simulink model "robot_capteur_etu"  (R2022a)
settings: Solver=VariableStepAuto  StartTime=0.0  StopTime=10.0  RelTol=1e-3
values from neighbouring files (symbols this model uses):
  K = -place(A, B, poles)    [matrices.m]    (also in sensibilite_parametre.m = [0.6700, 19.9053, 1.0747, 1.9614]; simu_robot_etu.m = [0.6700, 19.9055, 1.0747, 1.9614])
  ue = 0    [sensibilite_parametre.m]    (also in simu_robot_etu.m)
  x0 = [0 pi/10 0 0]'    [sensibilite_parametre.m]    (also in simu_robot_etu.m)
  xe = [0 0 0 0]'    [sensibilite_parametre.m]    (also in simu_robot_etu.m)
settings Model: Creator=nauchere  LastModifiedBy=nauchere

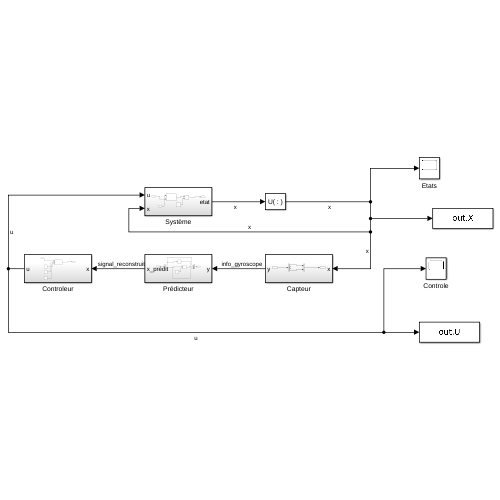
[thumbnail: Simulink's stored preview of the top-level diagram]
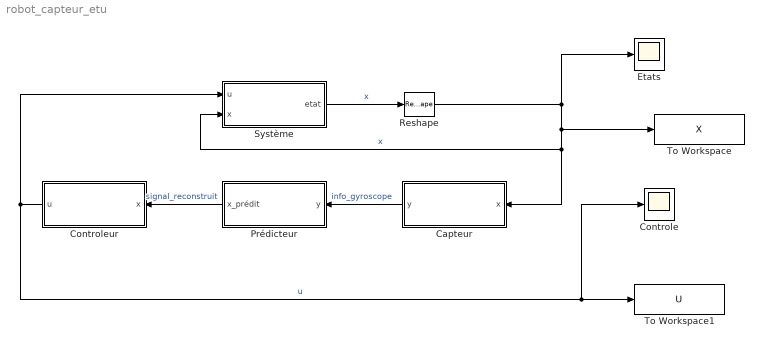
== system robot_capteur_etu ==
  Capteur : Subsystem
  Controle : Scope
  Controleur : Subsystem
  Etats : Scope
  Prédicteur : Subsystem
  Reshape : Reshape
  Système : Subsystem
  To Workspace : ToWorkspace  VariableName=X  SaveFormat=Timeseries  SampleTime=-1
  To Workspace1 : ToWorkspace  VariableName=U  SaveFormat=Timeseries  SampleTime=-1
  wires:
  Controleur/1(u) -> Système/1(u), Controle/1, To Workspace1/1  "u"
  Prédicteur/1(x_prédit) -> Controleur/1(x)  "signal_reconstruit"
  Capteur/1(y) -> Prédicteur/1(y)  "info_gyroscope"
  Reshape/1 -> Système/2(x), Capteur/1(x), To Workspace/1, Etats/1  "x"
  Système/1(etat) -> Reshape/1  "x"

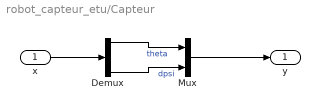
== system robot_capteur_etu/Capteur ==
  x : Inport
  Demux : Demux
  Mux : Mux  Inputs=2
  y : Outport
  wires:
  x/1 -> Demux/1
  Demux/1 -> Mux/1  "theta"
  Demux/4 -> Mux/2  "dpsi"
  Mux/1 -> y/1

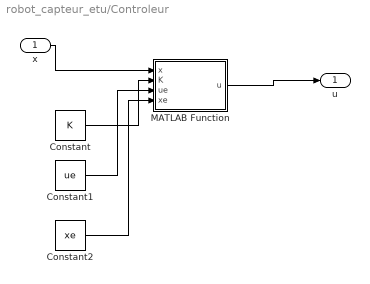
== system robot_capteur_etu/Controleur ==
  x : Inport
  Constant : Constant  Value=K  VectorParams1D=off
  Constant1 : Constant  Value=ue
  Constant2 : Constant  Value=xe  VectorParams1D=off
  MATLAB Function : MATLAB Function  TreatAsAtomicUnit=on
  u : Outport
  wires:
  Constant2/1 -> MATLAB Function/4(xe)
  MATLAB Function/1(u) -> u/1
  Constant/1 -> MATLAB Function/2(K)
  x/1 -> MATLAB Function/1(x)
  Constant1/1 -> MATLAB Function/3(ue)

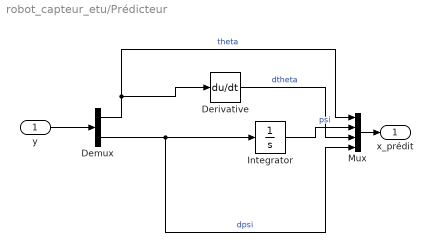
== system robot_capteur_etu/Prédicteur ==
  y : Inport
  Demux : Demux  Outputs=2
  Derivative : Derivative
  Integrator : Integrator
  Mux : Mux
  x_prédit : Outport
  wires:
  y/1 -> Demux/1
  Demux/2 -> Mux/4, Integrator/1  "dpsi"
  Mux/1 -> x_prédit/1
  Integrator/1 -> Mux/2  "psi"
  Demux/1 -> Derivative/1, Mux/1  "theta"
  Derivative/1 -> Mux/3  "dtheta"

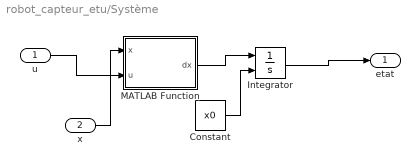
== system robot_capteur_etu/Système ==
  u : Inport
  x : Inport  Port=2
  Constant : Constant  Value=x0  VectorParams1D=off
  Integrator : Integrator  InitialConditionSource=external
  MATLAB Function : MATLAB Function  TreatAsAtomicUnit=on
  etat : Outport
  wires:
  u/1 -> MATLAB Function/2(u)
  x/1 -> MATLAB Function/1(x)
  Integrator/1 -> etat/1
  MATLAB Function/1(dx) -> Integrator/1
  Constant/1 -> Integrator/2

== matlab function robot_capteur_etu/Controleur/MATLAB Function ==
  data: x input; u output; K input; ue input; xe input
function u = fcn(x, K, ue, xe)

u = ue + K*(x - xe);
end

== matlab function robot_capteur_etu/Système/MATLAB Function ==
  data: x input; u input; dx output
function dx   = fonction( x, u)
%   Dynamic equations of motion of the segway on an axis.
%   Inputs: - x = [theta psi dtheta dpsi]
%               theta: average angle of the wheels      [rad]
%               psi: body pitch angle                   [rad]
%               dtheta: average velocity of the wheels  [rad/s]
%               dpsi: body pitch velocity               [rad/s]
%          - u: DC motor voltage (same value for both motors) [V]

    % State
    psi = x(2);
    dtheta = x(3);
    dpsi = x(4);

    % Parameters
    
    g = 9.81;           % gravity acceleration [m/sec^2]
    m = 0.03;           % wheel weight [kg]
    R = 0.04;           % wheel radius [m]
    Jw = m*R^2/2;       % wheel inertia moment [kg*m^2]
    M = 0.6;            % body weight [kg]
    H = 0.144;          % body height [m]
    L = H/2;            % distance of the center of mass from the wheel axle [m]
    Jpsi = M*L^2/3;     % body pitch inertia [kgm^2]
    Jm = 1e-5;          % DC motor inertia moment [kgm^2]
    Rm = 6.69;          % DC motor resistance [Ohm]
    Kb = 0.468;         % DC motor back EMF constant [Vsec/rad]
    Kt = 0.317;         % DC motor torque constant [Nm/A]
    n = 1;              % gear ratio
    fm = 0.0022;        % friction coefficient between body and DC motor
    fw = 0;             % friction coefficient between wheel and floor
    
    % Equations of motion
    c1 = (2*m+M)*R^2 + 2*Jw + 2*n^2*Jm;
    c2 = M*L*R*cos(psi) - 2*n^2*Jm;
    c3 = -M*L*R*dpsi^2*sin(psi);
    c4 = M*L^2 + Jpsi + 2*n^2*Jm;
    c5 = -M*g*L*sin(psi);

    alpha = Kt/Rm;
    beta = Kt*Kb/Rm + fm;

    Ftheta = alpha*(2*u) - 2*(beta+fw)*dtheta + 2*beta*dpsi;
    Fpsi = -alpha*(2*u) + 2*beta*dtheta - 2*beta*dpsi;

    ddtheta = (c4*c3 - c2*c5 + c4*Ftheta - c2*Fpsi)/(c4*c1 - c2^2);
    ddpsi = (Fpsi- c2*ddtheta - c5)/c4;
    dx = [dtheta dpsi ddtheta ddpsi]';

end
